simulink model "qpsk"  (R2018a)
settings: Solver=VariableStepAuto  StartTime=0.0  StopTime=4  RelTol=1e-3
libraries: commrandsrc3 x2, dsparch4 x2, commsink2 x1
settings Model: Creator=hp  LastModifiedBy=hp

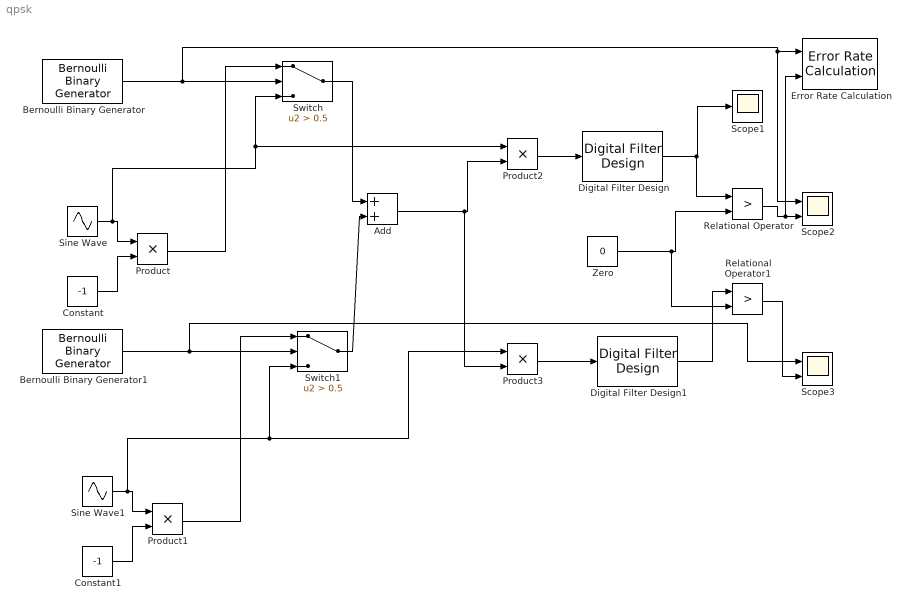
== system qpsk ==
  Add : Sum
  Bernoulli Binary Generator : commrandsrc3/Bernoulli Binary Generator  ProbabilityOfZero=0.5  SeedSource=Parameter  Seed=10  SampleTime=1  SamplesPerFrame=1  OutputDataType=double  SimulateUsing=Interpreted execution
  Bernoulli Binary Generator1 : commrandsrc3/Bernoulli Binary Generator  ProbabilityOfZero=0.5  SeedSource=Parameter  Seed=100  SampleTime=1  SamplesPerFrame=1  OutputDataType=double  SimulateUsing=Interpreted execution
  Constant : Constant  Value=-1
  Constant1 : Constant  Value=-1
  Digital Filter Design : dsparch4/Digital Filter Design  mwdsp_browser_bugfix_var=off
  Digital Filter Design1 : dsparch4/Digital Filter Design  mwdsp_browser_bugfix_var=off
  Error Rate Calculation : commsink2/Error Rate Calculation  N=0  st_delay=0  cp_mode=Entire frame  subframe=[]  PMode=Workspace  WsName=ErrorVec  RsMode2=off  stop=off  numErr=100  maxBits=1e6
  Product{,1..3} (4 alike) : Product
  Relational Operator : RelationalOperator  Operator=>  OutDataTypeStr=boolean  RndMeth=Simplest
  Relational Operator1 : RelationalOperator  Operator=>  OutDataTypeStr=boolean  RndMeth=Simplest
  Scope1 : Scope
  Scope2 : Scope  NumInputPorts=2
  Scope3 : Scope  NumInputPorts=2
  Sine Wave : Sin  Frequency=2*pi*2  SampleTime=0.001
  Sine Wave1 : Sin  Frequency=2*pi*2  Phase=180  SampleTime=0.001
  Switch : Switch  Criteria=u2 > Threshold  Threshold=0.5
  Switch1 : Switch  Criteria=u2 > Threshold  Threshold=0.5
  Zero : Constant  Value=0
  wires:
  Sine Wave/1 -> Product2/1, Switch/3, Product/1
  Constant/1 -> Product/2
  Bernoulli Binary Generator/1 -> Error Rate Calculation/1, Scope2/1, Switch/2
  Switch/1 -> Add/1
  Switch1/1 -> Add/2
  Sine Wave1/1 -> Product3/1, Switch1/3, Product1/1
  Constant1/1 -> Product1/2
  Bernoulli Binary Generator1/1 -> Scope3/1, Switch1/2
  Product/1 -> Switch/1
  Product1/1 -> Switch1/1
  Add/1 -> Product3/2, Product2/2
  Product2/1 -> Digital Filter Design/1
  Product3/1 -> Digital Filter Design1/1
  Digital Filter Design/1 -> Relational Operator/1, Scope1/1
  Digital Filter Design1/1 -> Relational Operator1/1
  Zero/1 -> Relational Operator1/2, Relational Operator/2
  Relational Operator/1 -> Error Rate Calculation/2, Scope2/2
  Relational Operator1/1 -> Scope3/2
